simulink model "simu"  (R2024a)
settings: Solver=VariableStepAuto  StartTime=0.0  StopTime=5  RelTol=1e-3
values from neighbouring files (symbols this model uses):
  k = 100    [Ode45.m]
  m = 10    [Ode45.m]
  r = 0.05    [Ode45.m]

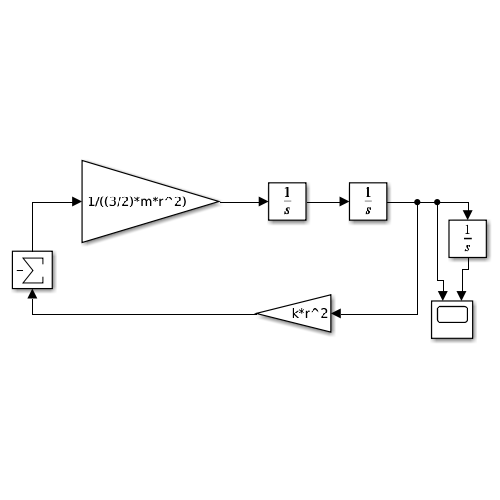
[thumbnail: Simulink's stored preview of the top-level diagram]
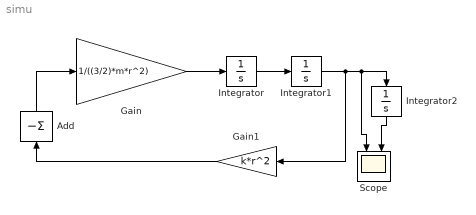
== system simu ==
  Add : Sum  Inputs=-
  Gain : Gain  Gain=1/((3/2)*m*r^2)
  Gain1 : Gain  Gain=k*r^2
  Integrator : Integrator
  Integrator1 : Integrator  InitialCondition=2
  Integrator2 : Integrator
  Scope : Scope  NumInputPorts=2
  wires:
  Add/1 -> Gain/1
  Gain/1 -> Integrator/1
  Integrator/1 -> Integrator1/1
  Gain1/1 -> Add/1
  Integrator1/1 -> Scope/1, Integrator2/1, Gain1/1
  Integrator2/1 -> Scope/2
